simulink model "sf_loop_scheduler"  (Simulink 7.6)
settings: Solver=FixedStepDiscrete  StartTime=0.0  StopTime=10  RelTol=1e-3
model workspace (MAT data in the model file):
  deltat : Simulink.Parameter (value not decoded)
settings Model: Creator=The MathWorks Inc.
settings SolverCC: InsertRTBMode=Auto
settings OptimizationCC: InitFltsAndDblsToZero=on
settings DebuggingCC: SaveWithParameterizedLinksMsg=none  SignalResolutionControl=TryResolveAllWithWarning  SolverPrmCheckMsg=none  InheritedTsInSrcMsg=none  MultiTaskDSMMsg=warning  MultiTaskCondExecSysMsg=none  StrictBusMsg=None
settings SFSimCC: SFSimEcho=off  SimParseCustomCode=off
settings RTWCC: IncludeERTFirstTime=on
settings GRTTargetCC: TargetFcnLib=ansi_tfl_tmw.mat

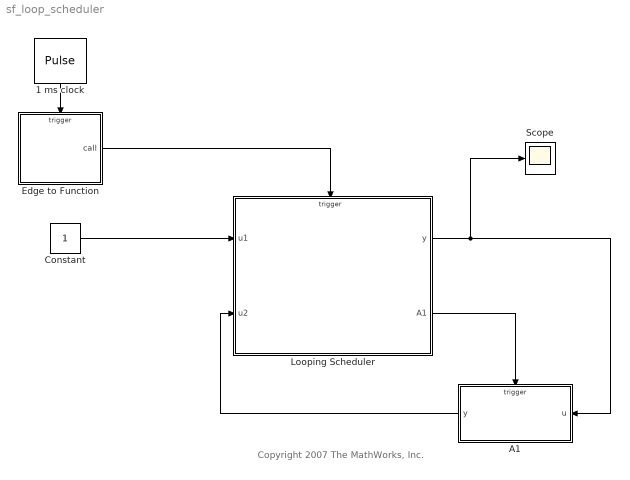
== system sf_loop_scheduler ==
  note: Copyright 2007 The MathWorks, Inc.
  1 ms clock : DiscretePulseGenerator  PulseType=Time based  Period=1  PulseWidth=10
  A1 : Subsystem  TreatAsAtomicUnit=on
  Constant : Constant
  "Edge to Function " : Stateflow chart  TreatAsAtomicUnit=on
  Looping Scheduler : Stateflow chart  TreatAsAtomicUnit=on
  Scope : Scope
      settings: TimeRange=10  YMin=0  YMax=100
  wires:
  Looping Scheduler/1(y) -> A1/1(u), Scope/1
  Looping Scheduler/2(A1) -> A1/Trigger
  A1/1(y) -> Looping Scheduler/2(u2)
  Constant/1 -> Looping Scheduler/1(u1)
  1 ms clock/1 -> "Edge to Function "/Trigger
  "Edge to Function "/1(call) -> Looping Scheduler/Trigger

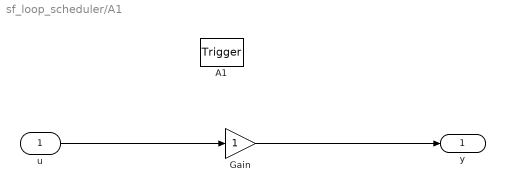
== system sf_loop_scheduler/A1 ==
  u : Inport
  A1 : TriggerPort  TriggerType=function-call
  Gain : Gain
  y : Outport
  wires:
  u/1 -> Gain/1
  Gain/1 -> y/1

== stateflow chart Looping Scheduler ==
  (junction 4) -> (junction 3) [order 1] : [i<=10]
      | {
      |  y = u1+u2;
      | send(A1);
      | i++;
      | }
  (junction 3) -> (junction 4)
  (default) -> (junction 3) : {i=1;}
  (junction 4) -> (junction 5) [order 2] : // done
  data: y output double; u1 input double; u2 input double; i local uint32
  events: A1 output FUNCTION_CALL_EVENT; call input FUNCTION_CALL_EVENT

== stateflow chart Edge to Function  ==
  (default) -> (junction 18) : {call;}
  events: edge input RISING_EDGE_EVENT; call output FUNCTION_CALL_EVENT
